simulink model "Tidal_Turbine_Power"  (R2023a)
settings: Solver=VariableStepAuto  StartTime=0.0  StopTime=10.0  RelTol=1e-3
settings Model: Creator=Aman  LastModifiedBy=Aman

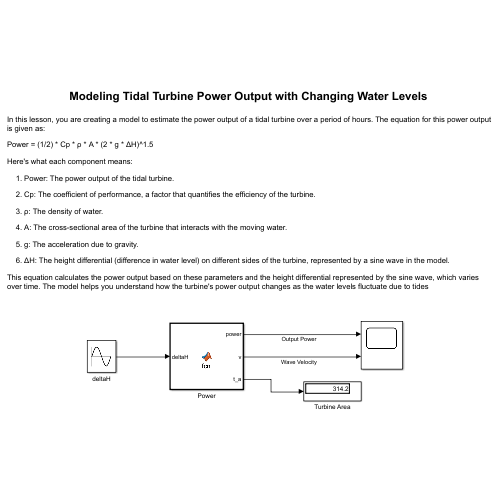
[thumbnail: Simulink's stored preview of the top-level diagram]
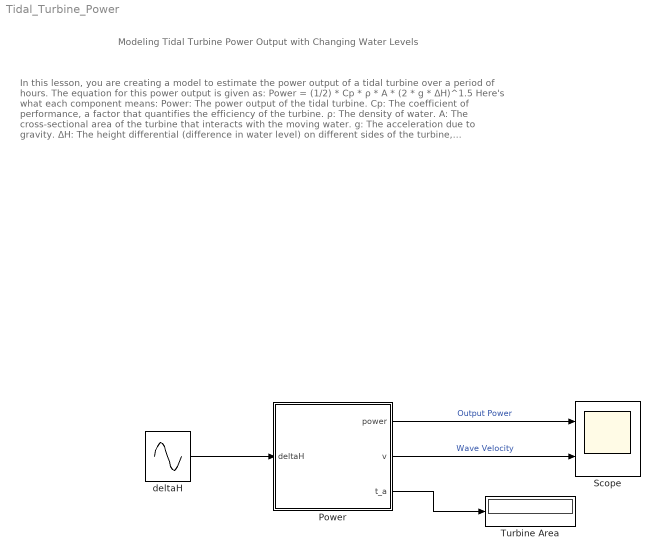
== system Tidal_Turbine_Power ==
  note: In this lesson, you are creating a model to estimate the power output of a tidal turbine over a period of hours. The equation for this power output is given as:
      | Power = (1/2) * Cp * ρ * A * (2 * g * ΔH)^1.5
      | Here's what each component means:
      | Power: The power output of the tidal turbine.
      | Cp: The coefficient of performance, a factor that quantifies the efficiency of the turbine.
      | ρ: The density of water.
      | A: The cross-sectional area of the turbine that interacts with the moving water.
      | g: The acceleration due to gravity.
      | ΔH: The height differential (difference in water level) on different sides of the turbine, represented by a sine wave in the model.
      | This equation calculates the power output based on these parameters and the height differential represented by the sine wave, which varies over time. The model helps you understand how the turbine's power output changes as the water levels fluctuate due to tides
  note: Modeling Tidal Turbine Power Output with Changing Water Levels
  Power : MATLAB Function  TreatAsAtomicUnit=on
  Scope : Scope  NumInputPorts=2
  Turbine Area : Display
  deltaH : Sin  Amplitude=.75  Frequency=0.5  SampleTime=0
  wires:
  Power/1(power) -> Scope/1  "Output Power"
  deltaH/1 -> Power/1(deltaH)
  Power/2(v) -> Scope/2  "Wave Velocity"
  Power/3(t_a) -> Turbine Area/1

== matlab function Tidal_Turbine_Power/Power ==
  data: deltaH input; power output; v output; t_a output
function [power, v, t_a] = fcn(deltaH)

Cp = 0.35; % Power coefficient
rho = 1000; % Density of water, kg/m^3
A = pi*10^2; % Area of turbine blade
turbineRadius = 10; % Radius of the turbine blade in meters
g = 9.81; % Acceleration of gravity, m/s^2


% Calculate the wave velocity
v = sqrt(2 * g * abs(deltaH));

% Calculate the cross-sectional area of the turbine
t_a = pi * turbineRadius^2;

% Replace the equation below with the correct equation for power
power = 0.5*Cp*rho*A*(2*g*abs(deltaH))^(3/2);
